simulink model "lista1_10"  (R2020b)
settings: Solver=VariableStepAuto  StartTime=0.0  StopTime=10  RelTol=1e-3
settings Model: Creator=lucas  LastModifiedBy=lucas

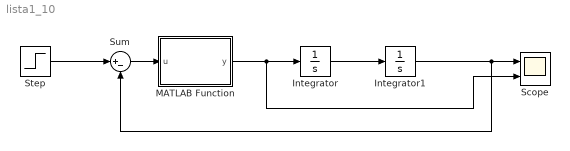
== system lista1_10 ==
  Integrator : Integrator
  Integrator1 : Integrator
  MATLAB Function : MATLAB Function  TreatAsAtomicUnit=on
  Scope : Scope  NumInputPorts=2
  Step : Step  Time=0  SampleTime=0
  Sum : Sum  Inputs=|+-
  wires:
  Step/1 -> Sum/1
  Sum/1 -> MATLAB Function/1(u)
  Integrator1/1 -> Scope/1, Sum/2
  Integrator/1 -> Integrator1/1
  MATLAB Function/1(y) -> Integrator/1, Scope/2

== matlab function lista1_10/MATLAB Function ==
  data: u input; y output
function y=sigmoid(u)
    y = 4/(1+exp(-100*u)) - 2;
end
